simulink model "dyn_braking_IM"  (R2015a)
settings: Solver=ode45  StartTime=0.0  StopTime=5  RelTol=1e-3
libraries: powerlib x12
settings Model: Creator=Debmalya Mukherjee  LastModifiedBy=debojyoti
settings OptimizationCC: ExpressionDepthLimit=2147483647
settings DebuggingCC: UnderspecifiedInitializationDetection=Classic  MergeDetectMultiDrivingBlocksExec=none  SolverPrmCheckMsg=warning  StateNameClashWarn=warning  StrictBusMsg=Warning
settings GRTTargetCC: CombineOutputUpdateFcns=off  GRTInterface=on

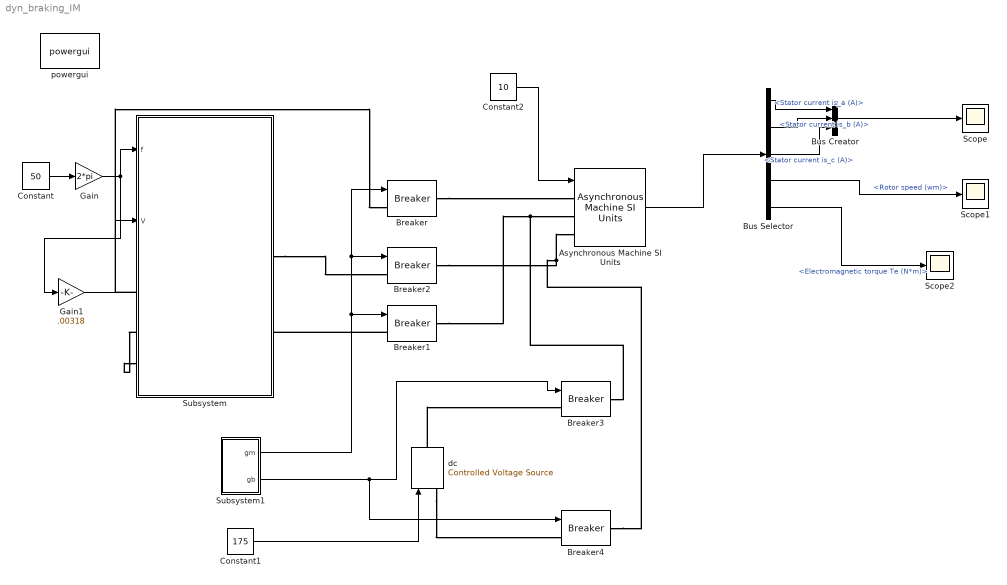
== system dyn_braking_IM ==
  Asynchronous Machine SI Units : powerlib/Machines/Asynchronous Machine SI Units  RotorType=Squirrel-cage  PresetModel=No  MechanicalLoad=Torque Tm  ShowDetailedParameters=on  ReferenceFrame=Rotor  Units=SI  MeasurementBus=off  NominalParameters=[10422.6 415 50]  Stator=[1.19 .008]  Rotor=[1.19 .008]  Cage1=[0.4155 0.002066]  Cage2=[0.4168 0.0003495]  Lm=.072  Mechanical=[.1 .03 2]  PolePairs=2  InitialConditions=[1 0 0 0 0 0 0 0]  SimulateSaturation=off  Saturation=[14.03593122, 27.81365428, 53.79336849, 72.68890987, 97.98006896, 148.6815601, 215.7428561, 302.9841135, 428.7778367 ; 230, 322, 414, 460, 506, 552, 598, 644, 690]  LoadFlowParameters=1492000  TsPowergui=0  TsBlock=-1  IterativeModel=Forward Euler  Pmec=1.492e+006
  Breaker{,1..4} (5 alike) : powerlib/Elements/Breaker  InitialState=0  SwitchingTimes="[ 1/60  5/60 ]"  External=on  BreakerResistance=0.01  SnubberResistance=1e6  SnubberCapacitance=inf  Measurements=None  MoreParameters=off  NoBreakLoop=off
  Bus Creator : BusCreator  Inputs=3
  Bus Selector : BusSelector  OutputSignals=Stator measurements.Stator current is_a (A),Stator measurements.Stator current is_b (A),Stator measurements.Stator current is_c (A),Mechanical.Rotor speed (wm),Mechanical.Electromagnetic torque Te (N*m)
  Constant : Constant  Value=50
  Constant1 : Constant  Value=175
  Constant2 : Constant  Value=10
  Gain : Gain  Gain=2*pi
  Gain1 : Gain  Gain=.00318
  Scope : Scope
      settings: YMin=-100  YMax=100
  Scope1 : Scope
      settings: YMin=-0.00325  YMax=0.00125
  Scope2 : Scope
      settings: YMin=-200  YMax=200  SaveName=ScopeData2
  Subsystem : Subsystem
  Subsystem1 : Subsystem
  dc : powerlib/Electrical Sources/Controlled Voltage Source  Initialize=on  Source_Type=AC  Amplitude=0  Phase=0  Frequency=0  Measurements=None
  powergui : powerlib/powergui  Priority=1  SimulationMode=Continuous  SolverType=Tustin/Backward Euler (TBE)  SampleTime=50e-6  frequency=60  SPID=off  DisableSnubberDevices=off  DisableRonSwitches=off  DisableVfSwitches=off  SwTol=0  DisplayEquations=off  Interpol=off  methode=off  Ts=0  FunctionMessages=off  echomessages=off  HookPort=off  EnableUseOfTLC=off  x0status=blocks  frequencyindice=50  Pbase=100e6  ErrMax=1e-4  Iterations=50  UnitsV=kV  UnitsW=MW  buscounter=0  RestoreLinks=warning  ResistiveCurrentMeasurement=off  Frange=[0:2:500]  Ylog=off  Xlog=on  ShowGrid=off  save=off  variable=ZData  structure=0  ZoomFFT=on  StartTime=0.0  cycles=1  DisplayStyle=1  fundamental=60  FreqAxis=off  MaxFrequency=1000  frequencyindicesteady=1  RmsSteady=1  display=off
  wires:
  Constant/1 -> Gain/1
  Gain/1 -> Subsystem/1(f), Gain1/1
  Gain1/1 -> Subsystem/2(V)
  Subsystem1/1(gm) -> Breaker/1, Breaker2/1, Breaker1/1
  Subsystem1/2(gb) -> Breaker3/1, Breaker4/1
  Constant1/1 -> dc/1
  Constant2/1 -> Asynchronous Machine SI Units/1
  Asynchronous Machine SI Units/1 -> Bus Selector/1
  Bus Selector/1 -> Bus Creator/1  "<Stator current is_a (A)>"
  Bus Selector/2 -> Bus Creator/2  "<Stator current is_b (A)>"
  Bus Selector/3 -> Bus Creator/3  "<Stator current is_c (A)>"
  Bus Creator/1 -> Scope/1
  Bus Selector/4 -> Scope1/1  "<Rotor speed (wm)>"
  Bus Selector/5 -> Scope2/1  "<Electromagnetic torque Te (N*m)>"
  connections:
  Subsystem/LConn1 -- Breaker/LConn1
  Breaker/RConn1 -- Asynchronous Machine SI Units/LConn1
  Breaker1/LConn1 -- Subsystem/LConn2
  Breaker1/RConn1 -- Asynchronous Machine SI Units/LConn2 -- Breaker3/RConn1
  Subsystem/RConn1 -- Breaker2/LConn1
  Breaker2/RConn1 -- Breaker4/RConn1 -- Asynchronous Machine SI Units/LConn3
  dc/RConn1 -- Breaker3/LConn1
  dc/LConn1 -- Breaker4/LConn1

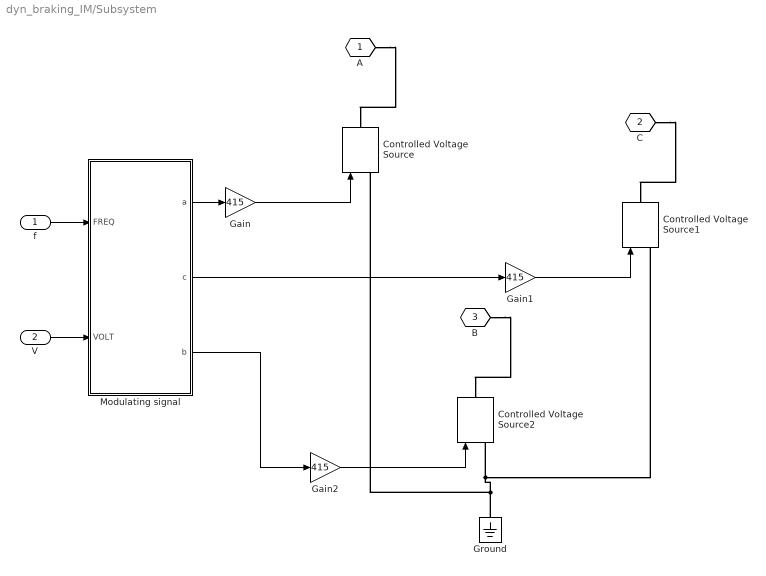
== system dyn_braking_IM/Subsystem ==
  f : Inport
  V : Inport  Port=2
  Controlled Voltage Source : powerlib/Electrical Sources/Controlled Voltage Source  Initialize=on  Source_Type=AC  Amplitude=0  Phase=0  Frequency=0  Measurements=None
  Controlled Voltage Source1 : powerlib/Electrical Sources/Controlled Voltage Source  Initialize=on  Source_Type=AC  Amplitude=0  Phase=0  Frequency=0  Measurements=None
  Controlled Voltage Source2 : powerlib/Electrical Sources/Controlled Voltage Source  Initialize=on  Source_Type=AC  Amplitude=0  Phase=0  Frequency=0  Measurements=None
  Gain : Gain  Gain=415
  Gain1 : Gain  Gain=415
  Gain2 : Gain  Gain=415
  Ground : powerlib/Elements/Ground  LConnTagsString=a
  Modulating signal : Subsystem
  A : PMIOPort  Tag=PMCPort  Port=1  Side=Left
  C : PMIOPort  Tag=PMCPort  Port=2  Side=Right
  B : PMIOPort  Tag=PMCPort  Port=3  Side=Left
  wires:
  V/1 -> Modulating signal/2(VOLT)
  f/1 -> Modulating signal/1(FREQ)
  Modulating signal/1(a) -> Gain/1
  Gain/1 -> Controlled Voltage Source/1
  Gain1/1 -> Controlled Voltage Source1/1
  Modulating signal/2(c) -> Gain1/1
  Gain2/1 -> Controlled Voltage Source2/1
  Modulating signal/3(b) -> Gain2/1
  connections:
  Controlled Voltage Source/LConn1 -- Ground/LConn1 -- Controlled Voltage Source2/LConn1 -- Controlled Voltage Source1/LConn1
  A/RConn1 -- Controlled Voltage Source/RConn1
  C/RConn1 -- Controlled Voltage Source1/RConn1
  B/RConn1 -- Controlled Voltage Source2/RConn1

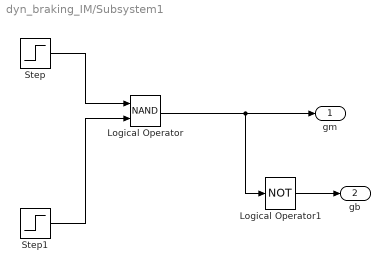
== system dyn_braking_IM/Subsystem1 ==
  Logical Operator : Logic  Operator=NAND  AllPortsSameDT=off  OutDataTypeStr=boolean
  Logical Operator1 : Logic  Operator=NOT  AllPortsSameDT=off  OutDataTypeStr=boolean
  Step : Step  Time=0  SampleTime=0
  Step1 : Step  Time=3.6  SampleTime=0
  gm : Outport
  gb : Outport  Port=2
  wires:
  Step/1 -> Logical Operator/1
  Step1/1 -> Logical Operator/2
  Logical Operator/1 -> gm/1, Logical Operator1/1
  Logical Operator1/1 -> gb/1

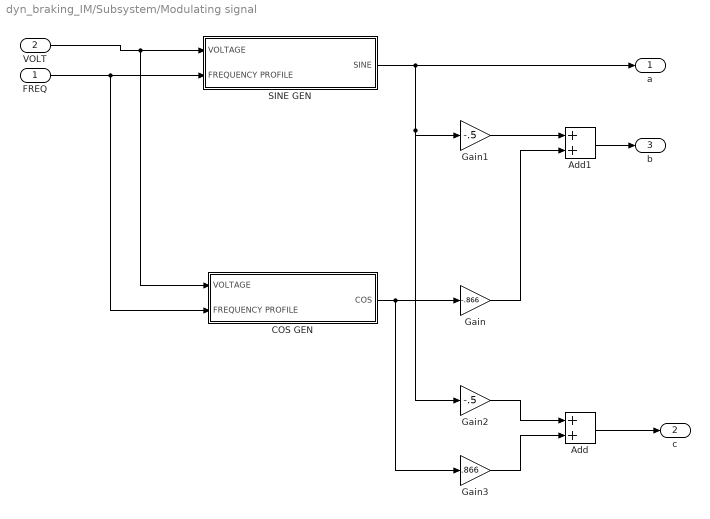
== system dyn_braking_IM/Subsystem/Modulating signal ==
  FREQ : Inport
  VOLT : Inport  Port=2
  Add : Sum
  Add1 : Sum
  COS GEN : Subsystem
  Gain : Gain  Gain=-.866
  Gain1 : Gain  Gain=-.5
  Gain2 : Gain  Gain=-.5
  Gain3 : Gain  Gain=.866
  SINE GEN : Subsystem
  a : Outport
  c : Outport  Port=2
  b : Outport  Port=3
  wires:
  FREQ/1 -> SINE GEN/2(FREQUENCY PROFILE), COS GEN/2(FREQUENCY PROFILE)
  VOLT/1 -> SINE GEN/1(VOLTAGE), COS GEN/1(VOLTAGE)
  SINE GEN/1(SINE) -> a/1, Gain1/1, Gain2/1
  Gain1/1 -> Add1/1
  Add1/1 -> b/1
  COS GEN/1(COS) -> Gain/1, Gain3/1
  Gain/1 -> Add1/2
  Gain3/1 -> Add/2
  Gain2/1 -> Add/1
  Add/1 -> c/1

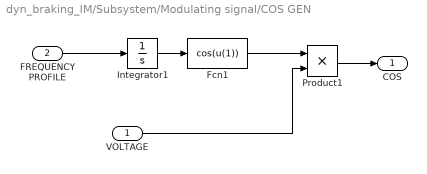
== system dyn_braking_IM/Subsystem/Modulating signal/COS GEN ==
  VOLTAGE : Inport
  FREQUENCY PROFILE : Inport  Port=2
  Fcn1 : Fcn  Expr=cos(u(1))
  Integrator1 : Integrator
  Product1 : Product  RndMeth=Zero
  COS : Outport
  wires:
  FREQUENCY PROFILE/1 -> Integrator1/1
  Integrator1/1 -> Fcn1/1
  Fcn1/1 -> Product1/1
  VOLTAGE/1 -> Product1/2
  Product1/1 -> COS/1

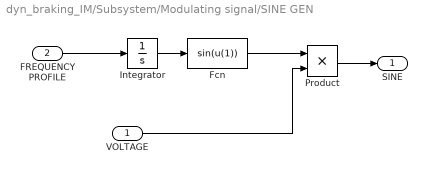
== system dyn_braking_IM/Subsystem/Modulating signal/SINE GEN ==
  VOLTAGE : Inport
  FREQUENCY PROFILE : Inport  Port=2
  Fcn : Fcn  Expr=sin(u(1))
  Integrator : Integrator
  Product : Product  RndMeth=Zero
  SINE : Outport
  wires:
  FREQUENCY PROFILE/1 -> Integrator/1
  Integrator/1 -> Fcn/1
  Fcn/1 -> Product/1
  VOLTAGE/1 -> Product/2
  Product/1 -> SINE/1
